simulink model "RHP_MIMO"  (R2015a)
settings: Solver=ode23s  StartTime=0.0  StopTime=10.0  RelTol=1e-3
values from neighbouring files (symbols this model uses):
  G_actual = zpk([(s-1)/(s+2) 4/(s+2); 4.5/(s+2) 2*(s-1)/(s+2)])    [mimo_rhpzero.m]
libraries: cstblocks x8
settings Model: Creator=dj  LastModifiedBy=dj

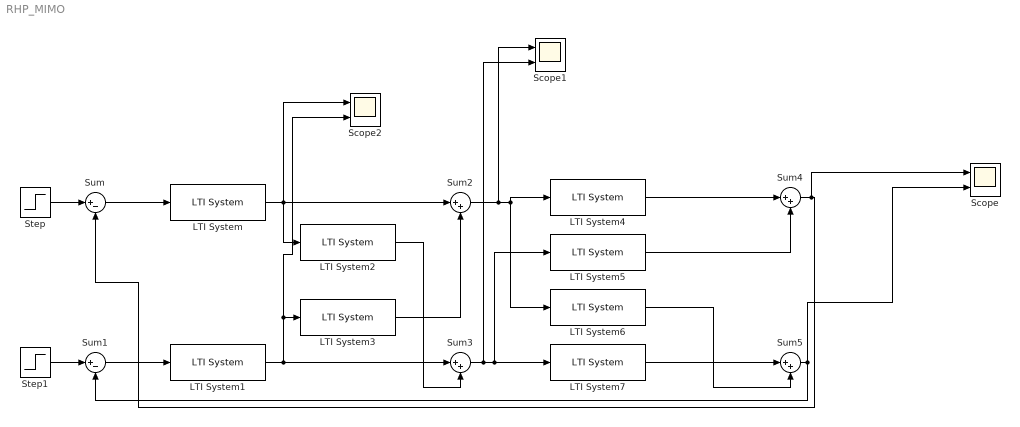
== system RHP_MIMO ==
  LTI System : cstblocks/LTI System  sys=Gc_11  IC=[]
  LTI System1 : cstblocks/LTI System  sys=Gc_22  IC=[]
  LTI System2 : cstblocks/LTI System  sys=Gc_12  IC=[]
  LTI System3 : cstblocks/LTI System  sys=Gc_21  IC=[]
  LTI System4 : cstblocks/LTI System  sys=G_actual(1,1)  IC=[]
  LTI System5 : cstblocks/LTI System  sys=G_actual(1,2)  IC=[]
  LTI System6 : cstblocks/LTI System  sys=G_actual(2,1)  IC=[]
  LTI System7 : cstblocks/LTI System  sys=G_actual(2,2)  IC=[]
  Scope : Scope  NumInputPorts=2
      settings: YMin=-5~-5  YMax=5~5
  Scope1 : Scope  NumInputPorts=2
      settings: YMin=-5~-5  YMax=5~5
  Scope2 : Scope  NumInputPorts=2
      settings: YMin=-5~-5  YMax=5~5  SaveName=ScopeData2
  Step : Step  SampleTime=0
  Step1 : Step  SampleTime=0
  Sum : Sum  Inputs=|+-
  Sum1 : Sum  Inputs=|+-
  Sum{2..5} (4 alike) : Sum  Inputs=|++
  wires:
  Sum1/1 -> LTI System1/1
  Sum/1 -> LTI System/1
  LTI System/1 -> Scope2/1, LTI System2/1, Sum2/1
  LTI System1/1 -> Scope2/2, LTI System3/1, Sum3/1
  LTI System3/1 -> Sum2/2
  LTI System2/1 -> Sum3/2
  Sum2/1 -> Scope1/1, LTI System6/1, LTI System4/1
  Sum3/1 -> Scope1/2, LTI System5/1, LTI System7/1
  LTI System7/1 -> Sum5/1
  LTI System4/1 -> Sum4/1
  LTI System5/1 -> Sum4/2
  LTI System6/1 -> Sum5/2
  Sum4/1 -> Scope/1, Sum/2
  Sum5/1 -> Scope/2, Sum1/2
  Step/1 -> Sum/1
  Step1/1 -> Sum1/1
